simulink model "circuito2"  (R2025a)
settings: Solver=VariableStepAuto  StartTime=0.0  StopTime=100  RelTol=1e-3  AbsTol=1e-3
libraries: fl_lib x22, nesl_utility x12
settings Model: Creator=Okuyt  LastModifiedBy=Okuyt
settings SolverCC: AutoScaleAbsTol=off  AlgebraicLoopSolver=TrustRegion  MaxZcPerStep=1.0
settings DebuggingCC: UnconnectedInputMsg=warning  UnconnectedOutputMsg=warning  UnconnectedLineMsg=warning  SymbolicDimsDataTypeCodeGenerationDiagnostic=none
settings ModelReferenceCC: EnableRefExpFcnMdlSchedulingChecks=on
settings SFSimCC: CustomCodeUndefinedFunction=UseInterfaceOnly
settings RTWCC: GPUComputeCapability=3.5  DLArmComputeVersion=19.05
settings SimscapeCC: SimscapeLogType=all  SimscapeLogSimulationStatistics=on  SimscapeLogDataHistory=10000.0

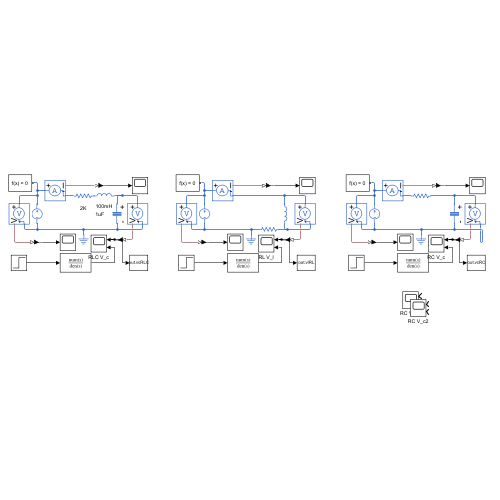
[thumbnail: Simulink's stored preview of the top-level diagram]
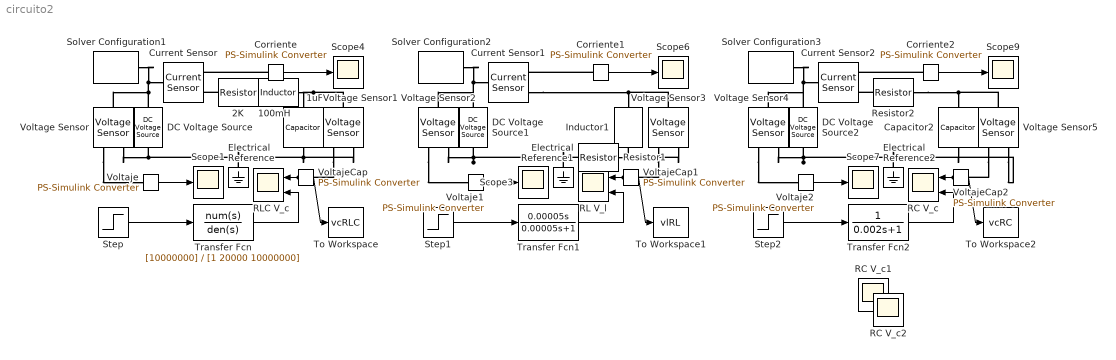
== system circuito2 ==
  100mH : fl_lib/Electrical/Electrical Elements/Inductor  l=100 mH  r=0 Ohm  g=1e-9 1/Ohm  i_specify=off  i_priority=None  i=0 A  i_nominal_specify=off  i_nominal_value=1  i_nominal_unit=A  v_specify=off  v_priority=None  v=0 V  v_nominal_specify=off  v_nominal_value=1  v_nominal_unit=V  i_L_specify=off  i_L_priority=High  i_L=0 A  i_L_nominal_specify=off  i_L_nominal_value=1  i_L_nominal_unit=A
  1uF : fl_lib/Electrical/Electrical Elements/Capacitor  c=1 uF  r=1e-6 Ohm  g=0 1/Ohm  i_specify=off  i_priority=None  i=0 A  i_nominal_specify=off  i_nominal_value=1  i_nominal_unit=A  v_specify=off  v_priority=None  v=0 V  v_nominal_specify=off  v_nominal_value=1  v_nominal_unit=V  vc_specify=off  vc_priority=High  vc=0 V  vc_nominal_specify=off  vc_nominal_value=1  vc_nominal_unit=V
  2K : fl_lib/Electrical/Electrical Elements/Resistor  R=2 kOhm  i_specify=off  i_priority=None  i=0 A  i_nominal_specify=off  i_nominal_value=1  i_nominal_unit=A  v_specify=off  v_priority=None  v=0 V  v_nominal_specify=off  v_nominal_value=1  v_nominal_unit=V
  Capacitor2 : fl_lib/Electrical/Electrical Elements/Capacitor  c=1 uF  r=1e-6 Ohm  g=0 1/Ohm  i_specify=off  i_priority=None  i=0 A  i_nominal_specify=off  i_nominal_value=1  i_nominal_unit=A  v_specify=off  v_priority=None  v=0 V  v_nominal_specify=off  v_nominal_value=1  v_nominal_unit=V  vc_specify=off  vc_priority=High  vc=0 V  vc_nominal_specify=off  vc_nominal_value=1  vc_nominal_unit=V
  Corriente : nesl_utility/PS-Simulink Converter  PhysicalDomain=network_engine_domain  SubClassName=ps_output  LeftPortType=input  RightPortType=output  PseudoPeriodic=off  Frequencies=[]  VectorFormat=inherit  Unit=inherit  AffineConversion=off
  Corriente1 : nesl_utility/PS-Simulink Converter  PhysicalDomain=network_engine_domain  SubClassName=ps_output  LeftPortType=input  RightPortType=output  PseudoPeriodic=off  Frequencies=[]  VectorFormat=inherit  Unit=inherit  AffineConversion=off
  Corriente2 : nesl_utility/PS-Simulink Converter  PhysicalDomain=network_engine_domain  SubClassName=ps_output  LeftPortType=input  RightPortType=output  PseudoPeriodic=off  Frequencies=[]  VectorFormat=inherit  Unit=inherit  AffineConversion=off
  Current Sensor : fl_lib/Electrical/Electrical Sensors/Current Sensor
  Current Sensor1 : fl_lib/Electrical/Electrical Sensors/Current Sensor
  Current Sensor2 : fl_lib/Electrical/Electrical Sensors/Current Sensor
  DC Voltage Source : fl_lib/Electrical/Electrical Sources/DC Voltage Source  v0=5 V
  DC Voltage Source1 : fl_lib/Electrical/Electrical Sources/DC Voltage Source  v0=5 V
  DC Voltage Source2 : fl_lib/Electrical/Electrical Sources/DC Voltage Source  v0=5 V
  Electrical Reference : fl_lib/Electrical/Electrical Elements/Electrical Reference
  Electrical Reference1 : fl_lib/Electrical/Electrical Elements/Electrical Reference
  Electrical Reference2 : fl_lib/Electrical/Electrical Elements/Electrical Reference
  Inductor1 : fl_lib/Electrical/Electrical Elements/Inductor  l=100 mH  r=0 Ohm  g=1e-9 1/Ohm  i_specify=off  i_priority=None  i=0 A  i_nominal_specify=off  i_nominal_value=1  i_nominal_unit=A  v_specify=off  v_priority=None  v=0 V  v_nominal_specify=off  v_nominal_value=1  v_nominal_unit=V  i_L_specify=off  i_L_priority=High  i_L=0 A  i_L_nominal_specify=off  i_L_nominal_value=1  i_L_nominal_unit=A
  RC V_c : Scope  NumInputPorts=2
      settings: Title=Funcion de transferencia vs Salida del circuito  ActiveDisplayYMinimum=-0.060650049082751956  ActiveDisplayYMaximum=4.9731070631350631  YLabel=Voltaje  DataLoggingVariableName=ScopeData6
  RC V_c1 : Scope  NumInputPorts=2
      settings: Title=Funcion de transferencia vs Salida del circuito  ActiveDisplayYMinimum=-3.53916868983982E-7  ActiveDisplayYMaximum=7.3529253989415817E-7  YLabel=Voltaje  DataLoggingVariableName=ScopeData8
  RC V_c2 : Scope  NumInputPorts=2
      settings: Title=Funcion de transferencia vs Salida del circuito  ActiveDisplayYMinimum=-0.060650049082751956  ActiveDisplayYMaximum=4.9731070631350631  YLabel=Voltaje  DataLoggingVariableName=ScopeData9
  RL V_l : Scope  NumInputPorts=2
      settings: Title=Funcion de transferencia vs Salida del circuito  ActiveDisplayYMinimum=-0.65199075700163123  ActiveDisplayYMaximum=7.4489023708659783  YLabel=Voltaje  DataLoggingVariableName=ScopeData3
  RLC V_c : Scope  NumInputPorts=2
      settings: Title=Funcion de transferencia vs Salida del circuito  ActiveDisplayYMinimum=-0.060650049082751956  ActiveDisplayYMaximum=4.9731070631350631  YLabel=Voltaje  DataLoggingVariableName=ScopeData2
  Resistor1 : fl_lib/Electrical/Electrical Elements/Resistor  R=2 kOhm  i_specify=off  i_priority=None  i=0 A  i_nominal_specify=off  i_nominal_value=1  i_nominal_unit=A  v_specify=off  v_priority=None  v=0 V  v_nominal_specify=off  v_nominal_value=1  v_nominal_unit=V
  Resistor2 : fl_lib/Electrical/Electrical Elements/Resistor  R=2 kOhm  i_specify=off  i_priority=None  i=0 A  i_nominal_specify=off  i_nominal_value=1  i_nominal_unit=A  v_specify=off  v_priority=None  v=0 V  v_nominal_specify=off  v_nominal_value=1  v_nominal_unit=V
  Scope{1,3..4,6..7,9} (6 alike) : Scope
      Scope1 settings: Title=Grafica de voltaje.  ActiveDisplayYMinimum=4  ActiveDisplayYMaximum=6  YLabel=Voltaje
      Scope3 settings: Title=Grafica de voltaje.  ActiveDisplayYMinimum=4  ActiveDisplayYMaximum=6  YLabel=Voltaje
      Scope4 settings: Title=Grafica de corriente  ActiveDisplayYMinimum=-0.0019993928048791867  ActiveDisplayYMaximum=0.0034772686897663217  YLabel=Intensidad
      Scope6 settings: Title=Grafica de corriente  ActiveDisplayYMinimum=-0.0019993928048791867  ActiveDisplayYMaximum=0.0034772686897663217  YLabel=Intensidad  DataLoggingVariableName=ScopeData4
      Scope7 settings: Title=Grafica de voltaje.  ActiveDisplayYMinimum=4  ActiveDisplayYMaximum=6  YLabel=Voltaje  DataLoggingVariableName=ScopeData5
      Scope9 settings: Title=Grafica de corriente  ActiveDisplayYMinimum=-0.00029355865758450358  ActiveDisplayYMaximum=0.0028103954050093891  YLabel=Intensidad  DataLoggingVariableName=ScopeData7
  Solver Configuration1 : nesl_utility/Solver Configuration  PhysicalDomain=network_engine_domain  SubClassName=solver  LeftPortType=input  RightPortType=generic  Tones=[]  Harmonics=[]  SimulateNoise=off  Profile=off  UseLocalSampling=off  EnableSwitchedLinearOptims=on  FrequencyDomain=off  UseCCode=off  RelTol=0.001  AbsTol=0.001  MinStep=1e-09  ToWorkspace=off  RevertToSquareIcSolve=off  NumHomotopyIterations=100  PhasorMode=off  PhasorModeNumHarmonics=1  ConsistencySolver=NEWTON_XTOL_AFTER_FTOL  IndexReductionMethod=DerivativeReplacement  DoDC=off  ResidualTolerance=1e-09  ConsistencyTolSource=GLOBAL  ConsistencyAbsTol=0.001  ConsistencyRelTol=0.001  ConsistencyTolFactor=0.001  UseLocalSolver=off  LocalSolverChoice=NE_BACKWARD_EULER_ADVANCER  ResolveIndetEquations=on  FunctionEvalNumThread=1  LocalSolverSampleTime=0.001  DoFixedCost=off  MaxNonlinIter=3  MaxModeIter=2  ComputeImpulses=off  ImpulseIterations=2  LinearAlgebra=auto  LinearAlgebraNumThread=0  EquationFormulation=NE_TIME_EF  DelaysMemoryBudget=1024  AutomaticFiltering=on  FilteringTimeConstant=0.001  PartitionStorageMethod=AS_NEEDED  PartitionMemoryBudget=1024  PartitionMethod=ROBUST  MultibodyUseLocalSolver=off  MultibodyLocalSolverChoice=ODE1  MultibodyLocalSolverSampleTime=0.001
  Solver Configuration2 : nesl_utility/Solver Configuration  PhysicalDomain=network_engine_domain  SubClassName=solver  LeftPortType=input  RightPortType=generic  Tones=[]  Harmonics=[]  SimulateNoise=off  Profile=off  UseLocalSampling=off  EnableSwitchedLinearOptims=on  FrequencyDomain=off  UseCCode=off  RelTol=0.001  AbsTol=0.001  MinStep=1e-09  ToWorkspace=off  RevertToSquareIcSolve=off  NumHomotopyIterations=100  PhasorMode=off  PhasorModeNumHarmonics=1  ConsistencySolver=NEWTON_XTOL_AFTER_FTOL  IndexReductionMethod=DerivativeReplacement  DoDC=off  ResidualTolerance=1e-09  ConsistencyTolSource=GLOBAL  ConsistencyAbsTol=0.001  ConsistencyRelTol=0.001  ConsistencyTolFactor=0.001  UseLocalSolver=off  LocalSolverChoice=NE_BACKWARD_EULER_ADVANCER  ResolveIndetEquations=on  FunctionEvalNumThread=1  LocalSolverSampleTime=0.001  DoFixedCost=off  MaxNonlinIter=3  MaxModeIter=2  ComputeImpulses=off  ImpulseIterations=2  LinearAlgebra=auto  LinearAlgebraNumThread=0  EquationFormulation=NE_TIME_EF  DelaysMemoryBudget=1024  AutomaticFiltering=on  FilteringTimeConstant=0.001  PartitionStorageMethod=AS_NEEDED  PartitionMemoryBudget=1024  PartitionMethod=ROBUST  MultibodyUseLocalSolver=off  MultibodyLocalSolverChoice=ODE1  MultibodyLocalSolverSampleTime=0.001
  Solver Configuration3 : nesl_utility/Solver Configuration  PhysicalDomain=network_engine_domain  SubClassName=solver  LeftPortType=input  RightPortType=generic  Tones=[]  Harmonics=[]  SimulateNoise=off  Profile=off  UseLocalSampling=off  EnableSwitchedLinearOptims=on  FrequencyDomain=off  UseCCode=off  RelTol=0.001  AbsTol=0.001  MinStep=1e-09  ToWorkspace=off  RevertToSquareIcSolve=off  NumHomotopyIterations=100  PhasorMode=off  PhasorModeNumHarmonics=1  ConsistencySolver=NEWTON_XTOL_AFTER_FTOL  IndexReductionMethod=DerivativeReplacement  DoDC=off  ResidualTolerance=1e-09  ConsistencyTolSource=GLOBAL  ConsistencyAbsTol=0.001  ConsistencyRelTol=0.001  ConsistencyTolFactor=0.001  UseLocalSolver=off  LocalSolverChoice=NE_BACKWARD_EULER_ADVANCER  ResolveIndetEquations=on  FunctionEvalNumThread=1  LocalSolverSampleTime=0.001  DoFixedCost=off  MaxNonlinIter=3  MaxModeIter=2  ComputeImpulses=off  ImpulseIterations=2  LinearAlgebra=auto  LinearAlgebraNumThread=0  EquationFormulation=NE_TIME_EF  DelaysMemoryBudget=1024  AutomaticFiltering=on  FilteringTimeConstant=0.001  PartitionStorageMethod=AS_NEEDED  PartitionMemoryBudget=1024  PartitionMethod=ROBUST  MultibodyUseLocalSolver=off  MultibodyLocalSolverChoice=ODE1  MultibodyLocalSolverSampleTime=0.001
  Step : Step  Time=0  After=5  SampleTime=0
  Step1 : Step  Time=0  After=5  SampleTime=0
  Step2 : Step  Time=0  After=5  SampleTime=0
  To Workspace : ToWorkspace  VariableName=vcRLC  SaveFormat=Timeseries  SampleTime=-1
  To Workspace1 : ToWorkspace  VariableName=vlRL  SaveFormat=Timeseries  SampleTime=-1
  To Workspace2 : ToWorkspace  VariableName=vcRC  SaveFormat=Timeseries  SampleTime=-1
  Transfer Fcn : TransferFcn  Numerator=[10000000]  Denominator=[1 20000 10000000]
  Transfer Fcn1 : TransferFcn  Numerator=[0.00005 0]  Denominator=[0.00005 1]
  Transfer Fcn2 : TransferFcn  Denominator=[0.002 1]
  Voltage Sensor{,1..5} (6 alike) : fl_lib/Electrical/Electrical Sensors/Voltage Sensor
  Voltaje : nesl_utility/PS-Simulink Converter  PhysicalDomain=network_engine_domain  SubClassName=ps_output  LeftPortType=input  RightPortType=output  PseudoPeriodic=off  Frequencies=[]  VectorFormat=inherit  Unit=inherit  AffineConversion=off
  Voltaje1 : nesl_utility/PS-Simulink Converter  PhysicalDomain=network_engine_domain  SubClassName=ps_output  LeftPortType=input  RightPortType=output  PseudoPeriodic=off  Frequencies=[]  VectorFormat=inherit  Unit=inherit  AffineConversion=off
  Voltaje2 : nesl_utility/PS-Simulink Converter  PhysicalDomain=network_engine_domain  SubClassName=ps_output  LeftPortType=input  RightPortType=output  PseudoPeriodic=off  Frequencies=[]  VectorFormat=inherit  Unit=inherit  AffineConversion=off
  VoltajeCap : nesl_utility/PS-Simulink Converter  PhysicalDomain=network_engine_domain  SubClassName=ps_output  LeftPortType=input  RightPortType=output  PseudoPeriodic=off  Frequencies=[]  VectorFormat=inherit  Unit=inherit  AffineConversion=off
  VoltajeCap1 : nesl_utility/PS-Simulink Converter  PhysicalDomain=network_engine_domain  SubClassName=ps_output  LeftPortType=input  RightPortType=output  PseudoPeriodic=off  Frequencies=[]  VectorFormat=inherit  Unit=inherit  AffineConversion=off
  VoltajeCap2 : nesl_utility/PS-Simulink Converter  PhysicalDomain=network_engine_domain  SubClassName=ps_output  LeftPortType=input  RightPortType=output  PseudoPeriodic=off  Frequencies=[]  VectorFormat=inherit  Unit=inherit  AffineConversion=off
  wires:
  Corriente/1 -> Scope4/1
  Step/1 -> Transfer Fcn/1
  Voltaje/1 -> Scope1/1
  Transfer Fcn/1 -> RLC V_c/2
  VoltajeCap/1 -> To Workspace/1, RLC V_c/1
  Transfer Fcn1/1 -> RL V_l/2
  Corriente1/1 -> Scope6/1
  Step1/1 -> Transfer Fcn1/1
  Voltaje1/1 -> Scope3/1
  VoltajeCap1/1 -> To Workspace1/1, RL V_l/1
  Transfer Fcn2/1 -> RC V_c/2
  Corriente2/1 -> Scope9/1
  Step2/1 -> Transfer Fcn2/1
  Voltaje2/1 -> Scope7/1
  VoltajeCap2/1 -> To Workspace2/1, RC V_c/1
  connections:
  2K/LConn1 -- Current Sensor/RConn2
  100mH/LConn1 -- 2K/RConn1
  Corriente/LConn1 -- Current Sensor/RConn1
  DC Voltage Source/LConn1 -- Voltage Sensor/LConn1 -- Solver Configuration1/RConn1 -- Current Sensor/LConn1
  1uF/RConn1 -- Electrical Reference/LConn1 -- Voltage Sensor/RConn2 -- DC Voltage Source/RConn1 -- Voltage Sensor1/RConn2
  Voltage Sensor/RConn1 -- Voltaje/LConn1
  100mH/RConn1 -- 1uF/LConn1 -- Voltage Sensor1/LConn1
  Voltage Sensor1/RConn1 -- VoltajeCap/LConn1
  DC Voltage Source1/RConn1 -- Resistor1/LConn1 -- Electrical Reference1/LConn1 -- Voltage Sensor2/RConn2
  Current Sensor1/LConn1 -- DC Voltage Source1/LConn1 -- Voltage Sensor2/LConn1 -- Solver Configuration2/RConn1
  Voltage Sensor3/LConn1 -- Current Sensor1/RConn2 -- Inductor1/LConn1
  Voltage Sensor2/RConn1 -- Voltaje1/LConn1
  Voltage Sensor3/RConn1 -- VoltajeCap1/LConn1
  Corriente1/LConn1 -- Current Sensor1/RConn1
  DC Voltage Source2/RConn1 -- Capacitor2/RConn1 -- Voltage Sensor5/RConn2 -- Electrical Reference2/LConn1 -- Voltage Sensor4/RConn2
  Voltage Sensor5/LConn1 -- Resistor2/RConn1 -- Capacitor2/LConn1
  Current Sensor2/LConn1 -- DC Voltage Source2/LConn1 -- Voltage Sensor4/LConn1 -- Solver Configuration3/RConn1
  Resistor2/LConn1 -- Current Sensor2/RConn2
  Voltage Sensor4/RConn1 -- Voltaje2/LConn1
  Voltage Sensor5/RConn1 -- VoltajeCap2/LConn1
  Corriente2/LConn1 -- Current Sensor2/RConn1
  Voltage Sensor3/RConn2 -- Inductor1/RConn1 -- Resistor1/RConn1
